simulink model "ExampleSelectorMinimumBlock"  (R2024a)
settings: Solver=VariableStepAuto  StartTime=0.0  StopTime=10.0  RelTol=1e-3
libraries: dspstat3 x1
settings Model: Creator=sonph  LastModifiedBy=sonph

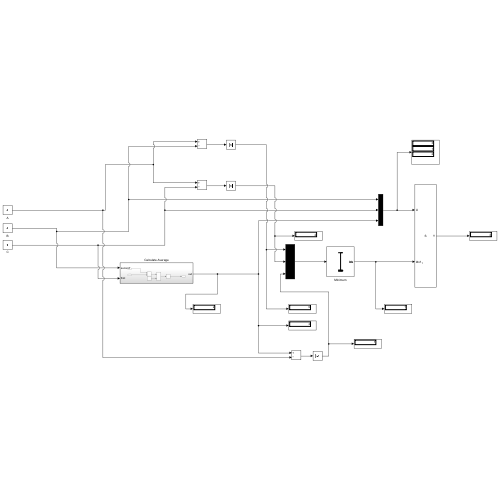
[thumbnail: Simulink's stored preview of the top-level diagram]
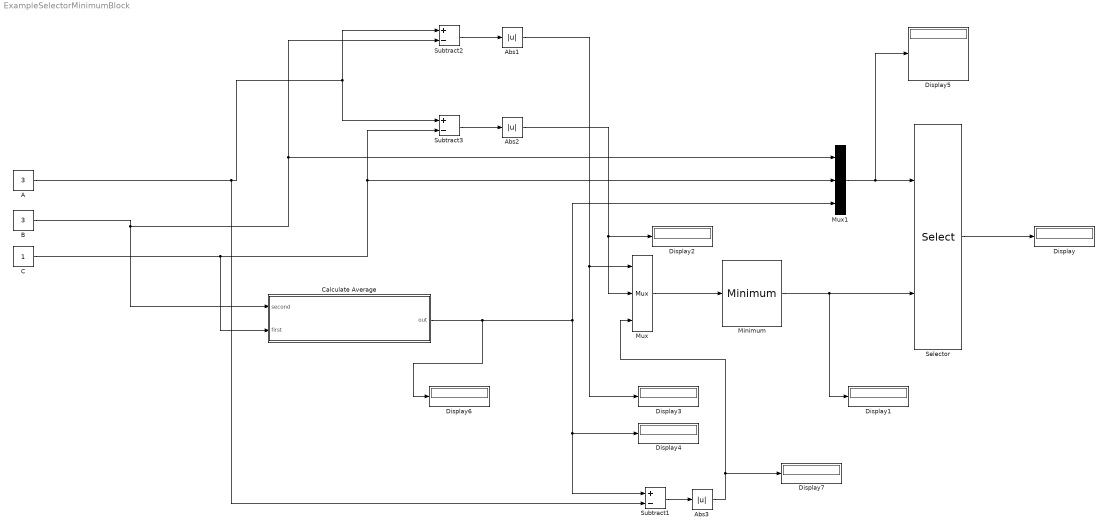
== system ExampleSelectorMinimumBlock ==
  A : Constant  Value=3  SampleTime=-1
  Abs1 : Abs  SaturateOnIntegerOverflow=off
  Abs2 : Abs  SaturateOnIntegerOverflow=off
  Abs3 : Abs  SaturateOnIntegerOverflow=off
  B : Constant  Value=3  SampleTime=-1
  C : Constant  SampleTime=-1
  Calculate Average : Subsystem
  Display{,1..7} (8 alike) : Display
  Minimum : dspstat3/Minimum  operation=minimum  fcn=Index  indexBase=One  operateOver=Each column  Dimension=1  InputProcessing=Columns as channels (frame based)  reset=None  roiEnable=off  roiType=Rectangles  roiPortion=Entire ROI  roiOutput=Individual statistics for each ROI  roiFlag=off  roundingMode=Floor  overflowMode=off
      settings: LibrarySourceBlock=dsphdlsupportstat/Minimum
  Mux : Mux  Inputs=3
  Mux1 : Mux  Inputs=3
  Selector : Selector  InputPortWidth=3  IndexOptions=Starting index (port)  Indices=[1 3]  OutputSizes=1
  Subtract1 : Sum  Inputs=+-
  Subtract2 : Sum  Inputs=+-
  Subtract3 : Sum  Inputs=+-
  wires:
  Mux/1 -> Minimum/1
  Mux1/1 -> Display5/1, Selector/1
  Minimum/1 -> Display1/1, Selector/2
  A/1 -> Subtract1/2, Subtract3/1, Subtract2/1
  Abs2/1 -> Display2/1, Mux/2
  Subtract2/1 -> Abs1/1
  Subtract3/1 -> Abs2/1
  B/1 -> Calculate Average/1(second), Mux1/1, Subtract2/2
  Abs1/1 -> Display3/1, Mux/1
  C/1 -> Mux1/2, Subtract3/2, Calculate Average/2(first)
  Calculate Average/1(out) -> Display6/1, Subtract1/1, Display4/1, Mux1/3
  Selector/1 -> Display/1
  Subtract1/1 -> Abs3/1
  Abs3/1 -> Mux/3, Display7/1

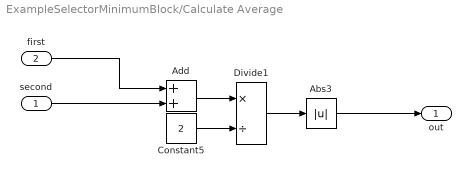
== system ExampleSelectorMinimumBlock/Calculate Average ==
  second : Inport
  first : Inport  Port=2
  Abs3 : Abs  SaturateOnIntegerOverflow=off
  Add : Sum
  Constant5 : Constant  Value=2
  Divide1 : Product  Inputs=*/
  out : Outport
  wires:
  second/1 -> Add/2
  Divide1/1 -> Abs3/1
  Constant5/1 -> Divide1/2
  Abs3/1 -> out/1
  first/1 -> Add/1
  Add/1 -> Divide1/1
